simulink model "sampleModel2046"  (R2023a)
settings: Solver=VariableStepAuto  StartTime=0.0  StopTime=10.0  RelTol=1e-3
libraries: hdlsllib x5, simulink x4
settings Model: Creator=user1  LastModifiedBy=user1

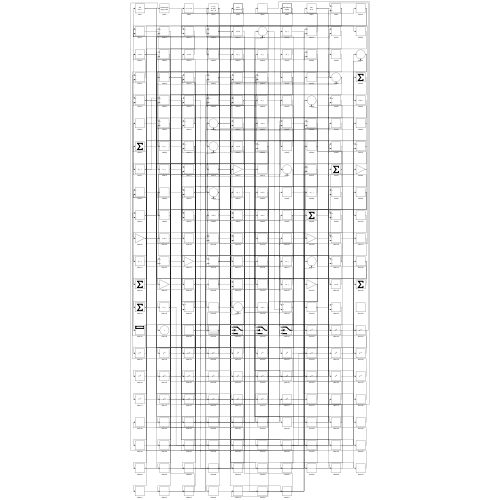
[thumbnail: Simulink's stored preview of the top-level diagram]
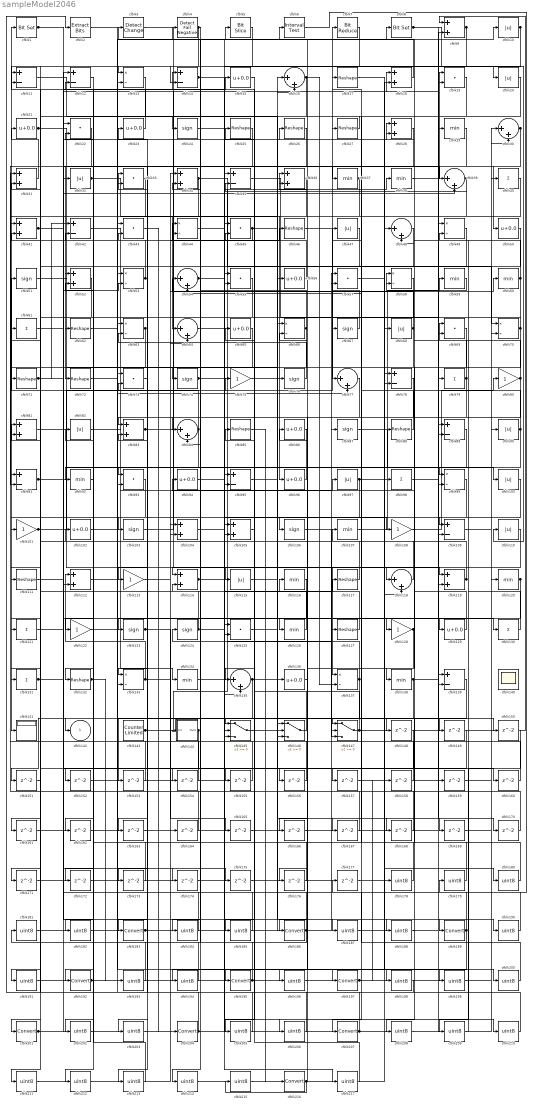
== system sampleModel2046 ==
  cfblk1 : simulink/Logic and Bit Operations/Bit Set  iBit=0
      settings: LibrarySourceBlock=|
      | hdlsllib/Logic and Bit
      | Operations/Bit Set
  cfblk{10,20,32,47,68,82,90,97,100,110,115} (11 alike) : Abs  SaturateOnIntegerOverflow=off
  cfblk{75,80,101,108,113,122,128} (7 alike) : Gain
  cfblk{15,21,23,50,56,65,86,94,96,102,129,136} (12 alike) : Bias  Bias=0.0  SaturateOnIntegerOverflow=off
  cfblk{24,51,67,74,76,87,103,106,123..124} (10 alike) : Signum
  cfblk{9,18,28,31,34,36,41,52,81,83,104..105,112,114,119} (15 alike) : Sum
  cfblk{29,37..38,59..60,92,107,116,120,126,134,138} (12 alike) : MinMax
  cfblk{11..12,14,35,42,78,89,91,95,109,139} (11 alike) : Sum  Inputs=+-
  cfblk{17,25..27,46,62,71..72,85,88,111,117,127,132} (14 alike) : Reshape
  cfblk{16,30,39,48,54,64,77,84,118,135} (10 alike) : Sum  Inputs=|++
  cfblk{40,61,79,98,121,130..131} (7 alike) : Sum  Inputs=+
  cfblk{19,22,33,43,45,55,57,69,73,93,125} (11 alike) : DotProduct  OutDataTypeStr=Inherit: Inherit via internal rule
  cfblk{13,44,49,53,58,63,66,70,99,133,137} (11 alike) : Product  Inputs=*/  RndMeth=Zero  SaturateOnIntegerOverflow=on
  cfblk140 : Scope
      settings: Floating=on
  cfblk141 : Display
  cfblk143 : hdlsllib/Sources/Counter Limited  uplimit=7  tsamp=-1
  cfblk144 : Subsystem
      settings: LibrarySourceBlock=|
      | hdlsllib/Ports &
      | Subsystems/Subsystem
  cfblk145 : Switch  SaturateOnIntegerOverflow=off  InputSameDT=off
  cfblk146 : Switch  SaturateOnIntegerOverflow=off  InputSameDT=off
  cfblk147 : Switch  SaturateOnIntegerOverflow=off  InputSameDT=off
  cfblk{148..177} (30 alike) : Delay  SampleTime=1
  cfblk{178..182,184..185,187..188,190..191,193..194,196,198..200,202..203,205..206,208..215,217} (30 alike) : DataTypeConversion  OutDataTypeStr=uint8  SaturateOnIntegerOverflow=off  RndMeth=Floor
  cfblk{183,186,189,192,195,197,201,204,207,216} (10 alike) : DataTypeConversion  SaturateOnIntegerOverflow=off  RndMeth=Floor
  cfblk2 : simulink/Logic and Bit Operations/Extract Bits  bitsToExtract=Upper half  numBits=8  bitIdxRange=[0 7]  outScalingMode=Preserve fixed-point scaling
      settings: LibrarySourceBlock=|
      | hdlsllib/Logic and Bit
      | Operations/Extract Bits
  cfblk3 : simulink/Logic and Bit Operations/Detect Change  vinit=0  OutDataTypeStr=boolean
      settings: LibrarySourceBlock=|
      | hdlsllib/Logic and Bit
      | Operations/Detect
      | Change
  cfblk4 : hdlsllib/Logic and Bit Operations/Detect Fall Negative  vinit=0  OutDataTypeStr=boolean
  cfblk5 : hdlsllib/Logic and Bit Operations/Bit Slice  lidx=7  ridx=0
  cfblk6 : hdlsllib/Logic and Bit Operations/Interval Test  IntervalClosedRight=on  uplimit=0.5  IntervalClosedLeft=on  lowlimit=-0.5  OutDataTypeStr=boolean
  cfblk7 : hdlsllib/Logic and Bit Operations/Bit Reduce  mode=AND
  cfblk8 : simulink/Logic and Bit Operations/Bit Set  iBit=0
      settings: LibrarySourceBlock=|
      | hdlsllib/Logic and Bit
      | Operations/Bit Set
  cfblk142 : Outport  VectorParamsAs1DForOutWhenUnconnected=off
  wires:
  cfblk39/1 -> cfblk96/1, cfblk35/2
  cfblk18/1 -> cfblk8/1
  cfblk108/1 -> cfblk80/1
  cfblk82/1 -> cfblk97/1
  cfblk93/1 -> cfblk141/1
  cfblk133/1 -> cfblk112/1, cfblk64/2
  cfblk132/1 -> cfblk82/1, cfblk193/1
  cfblk21/1 -> cfblk100/1, cfblk39/1
  cfblk42/1 -> cfblk134/1
  cfblk119/1 -> cfblk114/1, cfblk61/1
  cfblk143/1 -> cfblk36/1, cfblk75/1
  cfblk33/1 -> cfblk142/1
  cfblk40/1 -> cfblk101/1
  cfblk87/1 -> cfblk99/1
  cfblk38/1 -> cfblk19/1
  cfblk8/1 -> cfblk110/1, cfblk170/1
  cfblk126/1 -> cfblk33/1
  cfblk29/1 -> cfblk72/1
  cfblk63/1 -> cfblk131/1, cfblk71/1
  cfblk3/1 -> cfblk99/2
  cfblk90/1 -> cfblk122/1, cfblk127/1, cfblk54/2, cfblk196/1
  cfblk48/1 -> cfblk147/1
  cfblk83/1 -> cfblk137/1, cfblk46/1
  cfblk69/1 -> cfblk112/2
  cfblk7/1 -> cfblk41/1
  cfblk45/1 -> cfblk42/2, cfblk190/1
  cfblk103/1 -> cfblk19/2
  cfblk59/1 -> cfblk58/1
  cfblk130/1 -> cfblk69/1
  cfblk35/1 -> cfblk69/2
  cfblk89/1 -> cfblk186/1
  cfblk101/1 -> cfblk7/1, cfblk39/2
  cfblk68/1 -> cfblk54/1, cfblk157/1
  cfblk120/1 -> cfblk123/1, cfblk166/1
  cfblk99/1 -> cfblk109/1
  cfblk52/1 -> cfblk121/1
  cfblk66/1 -> cfblk14/1, cfblk145/2, cfblk182/1
  cfblk107/1 -> cfblk59/1
  cfblk100/1 -> cfblk133/1
  cfblk55/1 -> cfblk201/1
  cfblk60/1 -> cfblk83/1, cfblk3/1
  cfblk123/1 -> cfblk164/1, cfblk165/1
  cfblk71/1 -> cfblk128/1, cfblk42/1
  cfblk74/1 -> cfblk206/1, cfblk217/1
  cfblk31/1 -> cfblk21/1
  cfblk113/1 -> cfblk60/1
  cfblk125/1 -> cfblk76/1
  cfblk67/1 -> cfblk27/1
  cfblk53/1 -> cfblk113/1, cfblk11/2
  cfblk30/1 -> cfblk50/1, cfblk103/1
  cfblk9/1 -> cfblk74/1, cfblk13/1
  cfblk114/1 -> cfblk4/1, cfblk135/2, cfblk130/1, cfblk38/1
  cfblk80/1 -> cfblk58/2, cfblk145/3
  cfblk51/1 -> cfblk146/1
  cfblk75/1 -> cfblk118/1
  cfblk32/1 -> cfblk136/1, cfblk77/2
  cfblk146/1 -> cfblk25/1
  cfblk111/1 -> cfblk18/1
  cfblk116/1 -> cfblk195/1
  cfblk84/1 -> cfblk51/1, cfblk172/1
  cfblk54/1 -> cfblk160/1, cfblk198/1
  cfblk41/1 -> cfblk155/1, cfblk156/1
  cfblk79/1 -> cfblk106/1, cfblk48/2
  cfblk46/1 -> cfblk77/1
  cfblk97/1 -> cfblk145/1, cfblk169/1
  cfblk117/1 -> cfblk107/1
  cfblk118/1 -> cfblk34/2
  cfblk109/1 -> cfblk40/1
  cfblk27/1 -> cfblk24/1
  cfblk72/1 -> cfblk115/1
  cfblk85/1 -> cfblk216/1
  cfblk23/1 -> cfblk1/1
  cfblk16/1 -> cfblk105/2, cfblk137/2
  cfblk92/1 -> cfblk132/1
  cfblk81/1 -> cfblk139/2
  cfblk144/1(Out1) -> cfblk161/1, cfblk162/1
  cfblk98/1 -> cfblk79/1
  cfblk131/1 -> cfblk81/1, cfblk175/1
  cfblk95/1 -> cfblk189/1
  cfblk88/1 -> cfblk47/1
  cfblk70/1 -> cfblk62/1, cfblk138/1
  cfblk138/1 -> cfblk109/2, cfblk194/1
  cfblk28/1 -> cfblk37/1
  cfblk128/1 -> cfblk147/3, cfblk176/1
  cfblk1/1 -> cfblk126/1, cfblk187/1
  cfblk124/1 -> cfblk117/1, cfblk31/2
  cfblk73/1 -> cfblk183/1
  cfblk2/1 -> cfblk197/1
  cfblk134/1 -> cfblk87/1
  cfblk25/1 -> cfblk91/2
  cfblk24/1 -> cfblk119/1
  cfblk86/1 -> cfblk125/2
  cfblk10/1 -> cfblk14/2, cfblk13/2
  cfblk12/1 -> cfblk192/1
  cfblk36/1 -> cfblk64/1
  cfblk91/1 -> cfblk56/1, cfblk53/2
  cfblk5/1 -> cfblk84/1
  cfblk34/1 -> cfblk70/1, cfblk173/1
  cfblk43/1 -> cfblk204/1
  cfblk147/1 -> cfblk9/1, cfblk11/1
  cfblk49/1 -> cfblk207/1
  cfblk96/1 -> cfblk93/1
  cfblk64/1 -> cfblk10/1
  cfblk22/1 -> cfblk52/1
  cfblk137/1 -> cfblk124/1, cfblk151/1
  cfblk135/1 -> cfblk28/1, cfblk153/1
  cfblk129/1 -> cfblk94/1
  cfblk105/1 -> cfblk45/2
  cfblk94/1 -> cfblk108/1
  cfblk127/1 -> cfblk6/1
  cfblk121/1 -> cfblk15/1
  cfblk76/1 -> cfblk63/2
  cfblk61/1 -> cfblk26/1
  cfblk14/1 -> cfblk20/1, cfblk129/1
  cfblk136/1 -> cfblk144/1(In1)
  cfblk19/1 -> cfblk92/1
  cfblk62/1 -> cfblk5/1
  cfblk20/1 -> cfblk67/1
  cfblk4/1 -> cfblk111/1, cfblk154/1
  cfblk58/1 -> cfblk135/1
  cfblk56/1 -> cfblk44/1
  cfblk11/1 -> cfblk66/1
  cfblk37/1 -> cfblk93/2, cfblk212/1
  cfblk112/1 -> cfblk148/1
  cfblk106/1 -> cfblk149/1
  cfblk44/1 -> cfblk150/1
  cfblk151/1 -> cfblk81/2
  cfblk65/1 -> cfblk152/1
  cfblk152/1 -> cfblk45/1
  cfblk153/1 -> cfblk53/1
  cfblk154/1 -> cfblk22/2
  cfblk155/1 -> cfblk105/1
  cfblk156/1 -> cfblk114/2
  cfblk157/1 -> cfblk139/1
  cfblk158/1 -> cfblk31/1
  cfblk159/1 -> cfblk30/1
  cfblk160/1 -> cfblk147/2
  cfblk161/1 -> cfblk133/2
  cfblk162/1 -> cfblk119/2
  cfblk77/1 -> cfblk163/1
  cfblk163/1 -> cfblk83/2
  cfblk164/1 -> cfblk91/1
  cfblk165/1 -> cfblk9/2
  cfblk166/1 -> cfblk18/2
  cfblk115/1 -> cfblk167/1
  cfblk167/1 -> cfblk34/1
  cfblk145/1 -> cfblk168/1
  cfblk168/1 -> cfblk146/2
  cfblk169/1 -> cfblk70/2
  cfblk170/1 -> cfblk84/2
  cfblk13/1 -> cfblk171/1
  cfblk171/1 -> cfblk48/1
  cfblk172/1 -> cfblk16/2
  cfblk173/1 -> cfblk52/2
  cfblk102/1 -> cfblk174/1
  cfblk174/1 -> cfblk125/1
  cfblk176/1 -> cfblk63/1
  cfblk17/1 -> cfblk178/1
  cfblk178/1 -> cfblk23/1
  cfblk6/1 -> cfblk179/1
  cfblk179/1 -> cfblk17/1
  cfblk57/1 -> cfblk180/1
  cfblk180/1 -> cfblk28/2
  cfblk181/1 -> cfblk57/1
  cfblk182/1 -> cfblk57/2
  cfblk183/1 -> cfblk146/3, cfblk16/1, cfblk33/2
  cfblk149/1 -> cfblk184/1
  cfblk184/1 -> cfblk73/1
  cfblk15/1 -> cfblk185/1
  cfblk185/1 -> cfblk73/2
  cfblk186/1 -> cfblk181/1, cfblk22/1
  cfblk187/1 -> cfblk89/1
  cfblk175/1 -> cfblk188/1
  cfblk188/1 -> cfblk89/2
  cfblk189/1 -> cfblk36/2, cfblk86/1, cfblk214/1
  cfblk190/1 -> cfblk95/1
  cfblk148/1 -> cfblk191/1
  cfblk191/1 -> cfblk95/2
  cfblk192/1 -> cfblk29/1, cfblk120/1
  cfblk193/1 -> cfblk12/1
  cfblk194/1 -> cfblk12/2
  cfblk195/1 -> cfblk44/2, cfblk88/1
  cfblk196/1 -> cfblk116/1
  cfblk197/1 -> cfblk159/1, cfblk158/1
  cfblk198/1 -> cfblk2/1
  cfblk177/1 -> cfblk199/1
  cfblk199/1 -> cfblk90/1
  cfblk122/1 -> cfblk200/1
  cfblk200/1 -> cfblk177/1
  cfblk201/1 -> cfblk32/1, cfblk68/1
  cfblk26/1 -> cfblk202/1
  cfblk202/1 -> cfblk55/1
  cfblk50/1 -> cfblk203/1
  cfblk203/1 -> cfblk55/2
  cfblk204/1 -> cfblk30/2, cfblk41/2
  cfblk110/1 -> cfblk205/1
  cfblk205/1 -> cfblk43/1
  cfblk206/1 -> cfblk43/2
  cfblk207/1 -> cfblk98/1, cfblk35/1
  cfblk139/1 -> cfblk208/1
  cfblk208/1 -> cfblk49/1
  cfblk150/1 -> cfblk209/1
  cfblk209/1 -> cfblk49/2
  cfblk104/1 -> cfblk210/1
  cfblk210/1 -> cfblk65/1
  cfblk47/1 -> cfblk211/1
  cfblk211/1 -> cfblk104/1
  cfblk212/1 -> cfblk104/2
  cfblk78/1 -> cfblk213/1
  cfblk213/1 -> cfblk102/1
  cfblk214/1 -> cfblk78/1
  cfblk215/1 -> cfblk78/2
  cfblk216/1 -> cfblk215/1, cfblk66/2, cfblk118/2
  cfblk217/1 -> cfblk85/1

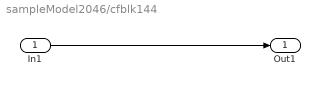
== system sampleModel2046/cfblk144 ==
  In1 : Inport
  Out1 : Outport
  wires:
  In1/1 -> Out1/1
